simulink model "SIM_nonlinear_mix_dis"  (R2016a)
settings: Solver=ode23t  SolverMode=SingleTasking  StartTime=0.0  StopTime=30  MaxStep=1e-4  RelTol=1e-3
undefined symbols (not defined in the file): A, B, input_dis, input_dis_time
libraries: dspsrcs4 x3
settings Model: Creator=edzel  LastModifiedBy=edzel
settings DataIOCC: ReturnWorkspaceOutputs=on
settings DebuggingCC: UnconnectedInputMsg=none  UnconnectedOutputMsg=none  UnconnectedLineMsg=none  SFUnexpectedBacktrackingDiag=error  SFNoUnconditionalDefaultTransitionDiag=error
settings ModelReferenceCC: EnableRefExpFcnMdlSchedulingChecks=off
settings SFSimCC: SimUseLocalCustomCode=on
settings RTWCC: Description=Generic Real-Time Target  RTWUseLocalCustomCode=on
settings GRTTargetCC: TargetLangStandard=C99 (ISO)
settings ConfigComp: CovMetricSettings=dwe  CovSaveCumulativeToWorkspaceVar=off  CovSaveSingleToWorkspaceVar=off  CovExternalEMLEnable=on

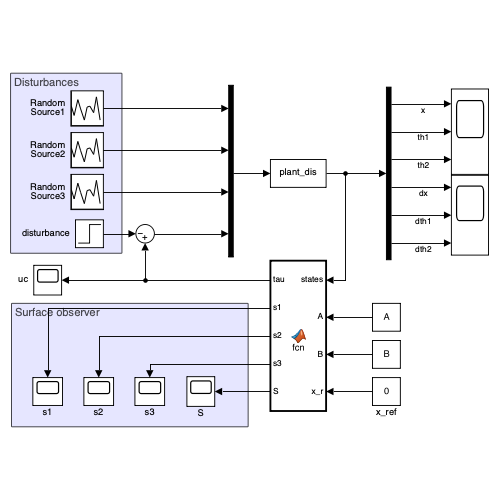
[thumbnail: Simulink's stored preview of the top-level diagram]
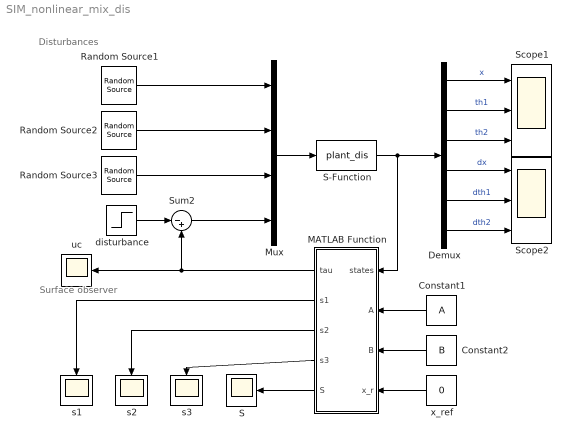
== system SIM_nonlinear_mix_dis ==
  note: Disturbances
  note: Surface observer
  Constant1 : Constant  Value=A
  Constant2 : Constant  Value=B
  Demux : Demux  Outputs=6
  MATLAB Function : MATLAB Function  TreatAsAtomicUnit=on
  Mux : Mux
  Random Source1 : dspsrcs4/Random Source  SrcType=Gaussian  NormMethod=Ziggurat  CltLength=12  MinVal=0  MaxVal=1  MeanVal=d1_mean  VarVal=d1_variance  RepMode=Specify seed  rawSeed=42  IsInherit=off  SampMode=Continuous  SampTime=1  SampFrame=1  DataType=Double  OutComplex=Real  OutputFrames=off
  Random Source2 : dspsrcs4/Random Source  SrcType=Gaussian  NormMethod=Ziggurat  CltLength=12  MinVal=0  MaxVal=1  MeanVal=d2_mean  VarVal=d2_variance  RepMode=Specify seed  rawSeed=42  IsInherit=off  SampMode=Continuous  SampTime=1  SampFrame=1  DataType=Double  OutComplex=Real  OutputFrames=off
  Random Source3 : dspsrcs4/Random Source  SrcType=Gaussian  NormMethod=Ziggurat  CltLength=12  MinVal=0  MaxVal=1  MeanVal=d3_mean  VarVal=d3_variance  RepMode=Specify seed  rawSeed=42  IsInherit=off  SampMode=Continuous  SampTime=1  SampFrame=1  DataType=Double  OutComplex=Real  OutputFrames=off
  S : Scope
  S-Function : S-Function  FunctionName=plant_dis  Parameters=CoeF1, CoeF2, CoeF3, theta1_rad, theta2_rad  SFunctionDeploymentMode=off  EnableBusSupport=off
  Scope1 : Scope  NumInputPorts=3
  Scope2 : Scope  NumInputPorts=3
  Sum2 : Sum  Inputs=|-+
  disturbance : Step  Time=input_dis_time  After=input_dis  SampleTime=0
  s1 : Scope
  s2 : Scope
  s3 : Scope
  uc : Scope
  x_ref : Constant  Value=0
  wires:
  Demux/5 -> Scope2/2  "dth1"
  Demux/3 -> Scope1/3  "th2"
  Demux/1 -> Scope1/1  "x"
  Demux/2 -> Scope1/2  "th1"
  Demux/4 -> Scope2/1  "dx"
  Demux/6 -> Scope2/3  "dth2"
  S-Function/1 -> MATLAB Function/1(states), Demux/1
  Constant1/1 -> MATLAB Function/2(A)
  Constant2/1 -> MATLAB Function/3(B)
  x_ref/1 -> MATLAB Function/4(x_r)
  MATLAB Function/3(s2) -> s2/1
  MATLAB Function/2(s1) -> s1/1
  MATLAB Function/5(S) -> S/1
  MATLAB Function/4(s3) -> s3/1
  MATLAB Function/1(tau) -> Sum2/2, uc/1
  disturbance/1 -> Sum2/1
  Sum2/1 -> Mux/4
  Mux/1 -> S-Function/1
  Random Source1/1 -> Mux/1
  Random Source2/1 -> Mux/2
  Random Source3/1 -> Mux/3

== matlab function SIM_nonlinear_mix_dis/MATLAB Function ==
  data: states input; tau output; A input; B input; x_r input; s1 output; s2 output; s3 output; S output
function [tau, s1, s2, s3, S] = fcn(states, A, B, x_r)

c1 = 2;       % 2
c2 = 5;         % 5
c3 = 1.3;       % 1.6 - 1.7？

alpha = 3;    % 1.5
beta =  8.8;     % 4.4
gamma = 5.4;    % 2.7

eta = 0.005;    % 0.005
k = 10;         % 20

x = states(1);
th1 = states(2);
th2 = states(3);

dx = states(4);
dth1 = states(5);
dth2 = states(6);

s1 = c1 * th1 + dth1;
s2 = c2 * th2 + dth2;
s3 = c3 * (x-x_r) + dx;

b1 = B(5, 1);
b2 = B(6, 1);
b3 = B(4, 1);

S = alpha * s1 + beta * s2 + gamma * s3;

% ueq1 = -(c1*dth1 + A(5,2)*th1 + A(5,3)*th2)/b1;
b1ueq1 = -(c1*dth1 + A(5,2)*th1 + A(5,3)*th2);

% ueq2 = -(c2*dth2 + A(6,2)*th1 + A(6,3)*th2)/b2;
b2ueq2 = -(c2*dth2 + A(6,2)*th1 + A(6,3)*th2);

% ueq3 = -(c3*dx + A(4,2)*th1 + A(4,3)*th2)/b3;
b3ueq3 = -(c3*dx + A(4,2)*th1 + A(4,3)*th2);

den = alpha * b1 + beta * b2 + gamma * b3;

u = (alpha*b1ueq1 + beta*b2ueq2 + gamma*b3ueq3 - eta*sign(S) -k*S) / den;

tau = u;


% Current advantage for SMC over LQR: better response at a cost of larger 
% angle change, but with smaller input.
% Not ideal for any desired destination.
% Good comparison at x_ref = 0.
